simulink model "sewermodel_malmo_mechanistic"  (R2017a)
settings: Solver=ode45  StartTime=0.0  StopTime=18  RelTol=1e-3
values from neighbouring files (symbols this model uses):
  Tair = 11+273.15    (= 284.15)    [init_model_malmo.m]
  Tsoil = 8+273.15    (= 281.15)    [init_model_malmo.m]
undefined symbols (not defined in the file or in its folder): amp, freq, gwbias, gwtemp, inf_onoff, noise_onoff, noise_std, nreservoirs, phase
settings Model: Creator=ielsaagi  LastModifiedBy=ielsaagi
settings DataIOCC: OutputOption=SpecifiedOutputTimes  OutputTimes=[0:5/(24*60):18]

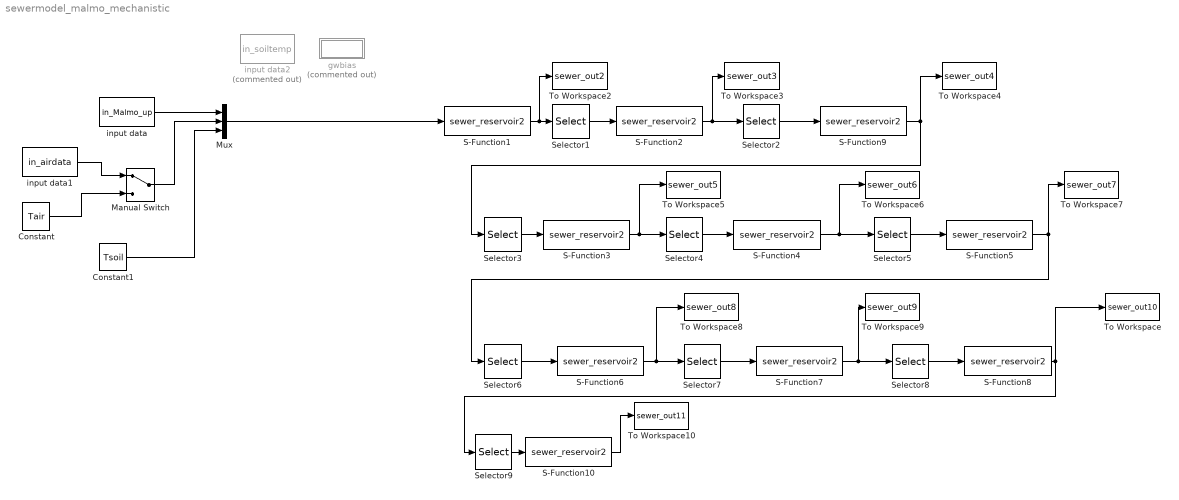
== system sewermodel_malmo_mechanistic ==
  Constant : Constant  Value=Tair
  Constant1 : Constant  Value=Tsoil
  Manual Switch : ManualSwitch
  Mux : Mux  Inputs=3
  S-Function1 : S-Function  FunctionName=sewer_reservoir2  Parameters=XINIT, DIM2, PARAM, Aratio, Siratio, Hratio,ONOFF  SFunctionDeploymentMode=off  EnableBusSupport=off
  S-Function10 : S-Function  FunctionName=sewer_reservoir2  Parameters=XINIT, DIM11, PARAM, Aratio, Siratio, Hratio,ONOFF  SFunctionDeploymentMode=off  EnableBusSupport=off
  S-Function2 : S-Function  FunctionName=sewer_reservoir2  Parameters=XINIT, DIM3, PARAM, Aratio, Siratio, Hratio,ONOFF  SFunctionDeploymentMode=off  EnableBusSupport=off
  S-Function3 : S-Function  FunctionName=sewer_reservoir2  Parameters=XINIT, DIM5, PARAM, Aratio, Siratio, Hratio,ONOFF  SFunctionDeploymentMode=off  EnableBusSupport=off
  S-Function4 : S-Function  FunctionName=sewer_reservoir2  Parameters=XINIT, DIM6, PARAM, Aratio, Siratio, Hratio,ONOFF  SFunctionDeploymentMode=off  EnableBusSupport=off
  S-Function5 : S-Function  FunctionName=sewer_reservoir2  Parameters=XINIT, DIM7, PARAM, Aratio, Siratio, Hratio,ONOFF  SFunctionDeploymentMode=off  EnableBusSupport=off
  S-Function6 : S-Function  FunctionName=sewer_reservoir2  Parameters=XINIT, DIM8, PARAM, Aratio, Siratio, Hratio,ONOFF  SFunctionDeploymentMode=off  EnableBusSupport=off
  S-Function7 : S-Function  FunctionName=sewer_reservoir2  Parameters=XINIT, DIM9, PARAM, Aratio, Siratio, Hratio,ONOFF  SFunctionDeploymentMode=off  EnableBusSupport=off
  S-Function8 : S-Function  FunctionName=sewer_reservoir2  Parameters=XINIT, DIM10, PARAM, Aratio, Siratio, Hratio,ONOFF  SFunctionDeploymentMode=off  EnableBusSupport=off
  S-Function9 : S-Function  FunctionName=sewer_reservoir2  Parameters=XINIT, DIM4, PARAM, Aratio, Siratio, Hratio,ONOFF  SFunctionDeploymentMode=off  EnableBusSupport=off
  Selector{1..9} (9 alike) : Selector  InputPortWidth=19  IndexOptions=Index vector (dialog)  Indices=[1:10]  OutputSizes=1
  To Workspace : ToWorkspace  VariableName=sewer_out10  SampleTime=-1
  To Workspace10 : ToWorkspace  VariableName=sewer_out11  SampleTime=-1
  To Workspace2 : ToWorkspace  VariableName=sewer_out2  SampleTime=-1
  To Workspace3 : ToWorkspace  VariableName=sewer_out3  SampleTime=-1
  To Workspace4 : ToWorkspace  VariableName=sewer_out4  SampleTime=-1
  To Workspace5 : ToWorkspace  VariableName=sewer_out5  SampleTime=-1
  To Workspace6 : ToWorkspace  VariableName=sewer_out6  SampleTime=-1
  To Workspace7 : ToWorkspace  VariableName=sewer_out7  SampleTime=-1
  To Workspace8 : ToWorkspace  VariableName=sewer_out8  SampleTime=-1
  To Workspace9 : ToWorkspace  VariableName=sewer_out9  SampleTime=-1
  gwbias : Subsystem  Commented=on
  input data : FromWorkspace  VariableName=in_Malmo_up  OutDataTypeStr=double  SampleTime=5/(24*60)  Interpolate=off  OutputAfterFinalValue=Cyclic repetition
  input data1 : FromWorkspace  VariableName=in_airdata  OutDataTypeStr=double  SampleTime=5/(24*60)  Interpolate=off  OutputAfterFinalValue=Cyclic repetition
  input data2 : FromWorkspace  Commented=on  VariableName=in_soiltemp  OutDataTypeStr=double  SampleTime=5/(24*60)  Interpolate=off  OutputAfterFinalValue=Cyclic repetition
  wires:
  S-Function8/1 -> Selector9/1, To Workspace/1
  S-Function1/1 -> To Workspace2/1, Selector1/1
  S-Function2/1 -> Selector2/1, To Workspace3/1
  S-Function9/1 -> Selector3/1, To Workspace4/1
  S-Function3/1 -> Selector4/1, To Workspace5/1
  S-Function4/1 -> Selector5/1, To Workspace6/1
  S-Function5/1 -> Selector6/1, To Workspace7/1
  S-Function6/1 -> Selector7/1, To Workspace8/1
  S-Function7/1 -> To Workspace9/1, Selector8/1
  Selector2/1 -> S-Function9/1
  Selector3/1 -> S-Function3/1
  Selector4/1 -> S-Function4/1
  Selector5/1 -> S-Function5/1
  Selector6/1 -> S-Function6/1
  Selector7/1 -> S-Function7/1
  Selector8/1 -> S-Function8/1
  Selector1/1 -> S-Function2/1
  Selector9/1 -> S-Function10/1
  S-Function10/1 -> To Workspace10/1
  input data/1 -> Mux/1
  Constant1/1 -> Mux/3
  Mux/1 -> S-Function1/1
  Constant/1 -> Manual Switch/2
  input data1/1 -> Manual Switch/1
  Manual Switch/1 -> Mux/2

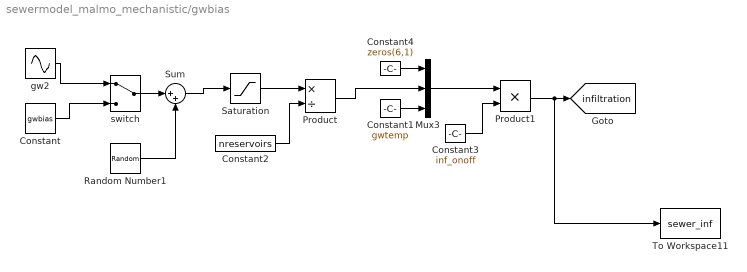
== system sewermodel_malmo_mechanistic/gwbias ==
  Constant : Constant  Value=gwbias
  Constant1 : Constant  Value=gwtemp
  Constant2 : Constant  Value=nreservoirs
  Constant3 : Constant  Value=inf_onoff
  Constant4 : Constant  Value=zeros(6,1)
  Mux3 : Mux  Inputs=3
  Product : Product  Inputs=*/
  Product1 : Product
  Random Number1 : RandomNumber  Variance=noise_onoff*power(gwbias*noise_std,2)  Seed=44  SampleTime=1/96
  Saturation : Saturate  UpperLimit=gwbias*5  LowerLimit=0
  Sum : Sum  Inputs=|++
  To Workspace11 : ToWorkspace  VariableName=sewer_inf  SampleTime=1/96
  gw2 : Sin  Amplitude=gwbias*amp  Bias=gwbias  Frequency=freq  Phase=phase  SampleTime=0
  "switch " : ManualSwitch
  tag scope: infiltration=global
  wires:
  Random Number1/1 -> Sum/2
  gw2/1 -> "switch "/1
  Constant/1 -> "switch "/2
  "switch "/1 -> Sum/1
  Sum/1 -> Saturation/1
  Constant4/1 -> Mux3/1
  Saturation/1 -> Product/1
  Constant1/1 -> Mux3/3
  Constant2/1 -> Product/2
  Product/1 -> Mux3/2
  Mux3/1 -> Product1/1
  Constant3/1 -> Product1/2
  Product1/1 -> To Workspace11/1, [infiltration]
